simulink model "untitled"  (R2023a)
settings: Solver=VariableStepAuto  StartTime=0.0  StopTime=10.0  RelTol=1e-3
settings Model: Creator=Пользователь  LastModifiedBy=Пользователь

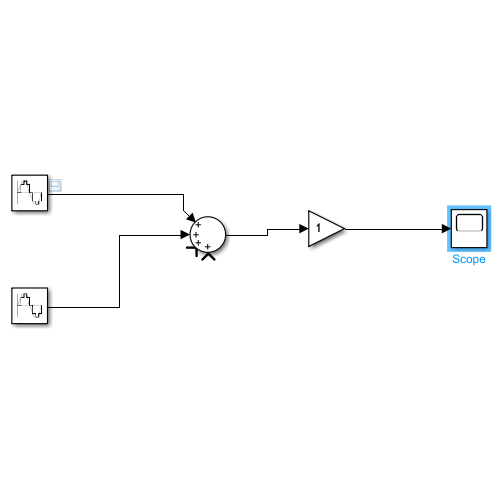
[thumbnail: Simulink's stored preview of the top-level diagram]
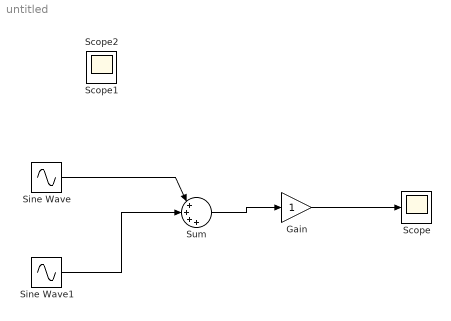
== system untitled ==
  Gain : Gain
  Scope : Scope
  Sine Wave : Sin  Amplitude=1:4  Frequency=5  Phase=-5  SampleTime=0.2
  Sine Wave1 : Sin  Amplitude=2  Frequency=5  Phase=-5  SampleTime=0.2
  Sum : Sum  Inputs=|++++
  Scope1 : Scope
  Scope2 : Scope
  wires:
  Sine Wave/1 -> Sum/1
  Sine Wave1/1 -> Sum/2
  Sum/1 -> Gain/1
  Gain/1 -> Scope/1
